simulink model "case4"  (R2024b)
settings: Solver=FixedStepAuto  StartTime=0  StopTime=1  FixedStep=1e-7  RelTol=1e-3
values from neighbouring files (symbols this model uses):
  SG_D_1_D = 0.01056    [IEEE9_case_parameters.m]    (also in case1_parameters.m; case2_parameters.m; case3_parameters.m; case4_parameters.m)
  SG_D_1_EnableSaturation = 0    [IEEE9_case_parameters.m]    (also in case1_parameters.m; case2_parameters.m; case3_parameters.m; case4_parameters.m)
  SG_D_1_f0 = 60    [IEEE9_case_parameters.m]    (also in case1_parameters.m; case2_parameters.m; case3_parameters.m; case4_parameters.m)
  SG_D_1_H = 7.5    [IEEE9_case_parameters.m]    (also in case1_parameters.m; case2_parameters.m; case3_parameters.m; case4_parameters.m)
  SG_D_1_K_A = 20    [IEEE9_case_parameters.m]    (also in case1_parameters.m; case2_parameters.m; case3_parameters.m; case4_parameters.m)
  SG_D_1_K_E = 1.000000e+1    (= 10)    [IEEE9_case_parameters.m]    (also in case1_parameters.m; case2_parameters.m; case3_parameters.m; case4_parameters.m)
  SG_D_1_K_F = 2.363    [IEEE9_case_parameters.m]    (also in case1_parameters.m; case2_parameters.m; case3_parameters.m; case4_parameters.m)
  SG_D_1_K_s = 0.5    [IEEE9_case_parameters.m]    (also in case1_parameters.m = 5; case2_parameters.m = 5; case3_parameters.m = 5; case4_parameters.m = 5)
  SG_D_1_R_a = 0.001088    [IEEE9_case_parameters.m]    (also in case1_parameters.m; case2_parameters.m; case3_parameters.m; case4_parameters.m)
  SG_D_1_S_A = 1    [IEEE9_case_parameters.m]    (also in case1_parameters.m; case2_parameters.m; case3_parameters.m; case4_parameters.m)
  SG_D_1_S_B = 0.103    [IEEE9_case_parameters.m]    (also in case1_parameters.m; case2_parameters.m; case3_parameters.m; case4_parameters.m)
  SG_D_1_S_N = 10.659857    [IEEE9_case_parameters.m]    (also in case1_parameters.m; case2_parameters.m; case3_parameters.m; case4_parameters.m)
  SG_D_1_SpeedPara = 200    [IEEE9_case_parameters.m]    (also in case1_parameters.m; case2_parameters.m; case3_parameters.m; case4_parameters.m)
  SG_D_1_T_0 = 0.720173    [IEEE9_case_parameters.m]    (also in case1_parameters.m = 0.755522; case2_parameters.m = 0.808931; case3_parameters.m = 0.869402; case4_parameters.m = 0.729316)
  SG_D_1_T_1 = 0.3    [IEEE9_case_parameters.m]    (also in case1_parameters.m; case2_parameters.m; case3_parameters.m; case4_parameters.m)
  SG_D_1_T_2 = 0.05    [IEEE9_case_parameters.m]    (also in case1_parameters.m; case2_parameters.m; case3_parameters.m; case4_parameters.m)
  SG_D_1_T_3 = 0.02    [IEEE9_case_parameters.m]    (also in case1_parameters.m; case2_parameters.m; case3_parameters.m; case4_parameters.m)
  SG_D_1_T_4 = 0.005    [IEEE9_case_parameters.m]    (also in case1_parameters.m; case2_parameters.m; case3_parameters.m; case4_parameters.m)
  SG_D_1_T_A = 0.02    [IEEE9_case_parameters.m]    (also in case1_parameters.m; case2_parameters.m; case3_parameters.m; case4_parameters.m)
  SG_D_1_T_dd = 8.000000e+0    (= 8)    [IEEE9_case_parameters.m]    (also in case1_parameters.m; case2_parameters.m; case3_parameters.m; case4_parameters.m)
  SG_D_1_T_ddd = 0.04    [IEEE9_case_parameters.m]    (also in case1_parameters.m; case2_parameters.m; case3_parameters.m; case4_parameters.m)
  SG_D_1_T_E = 0.314    [IEEE9_case_parameters.m]    (also in case1_parameters.m; case2_parameters.m; case3_parameters.m; case4_parameters.m)
  SG_D_1_T_F = 0.35    [IEEE9_case_parameters.m]    (also in case1_parameters.m; case2_parameters.m; case3_parameters.m; case4_parameters.m)
  SG_D_1_T_qd = 0.8    [IEEE9_case_parameters.m]    (also in case1_parameters.m; case2_parameters.m; case3_parameters.m; case4_parameters.m)
  SG_D_1_T_qdd = 0.02    [IEEE9_case_parameters.m]    (also in case1_parameters.m; case2_parameters.m; case3_parameters.m; case4_parameters.m)
  SG_D_1_T_speed = 0.1    [IEEE9_case_parameters.m]    (also in case1_parameters.m = 200; case2_parameters.m = 200; case3_parameters.m = 200; case4_parameters.m = 200)
  SG_D_1_T_w = 0.5    [IEEE9_case_parameters.m]    (also in case1_parameters.m; case2_parameters.m; case3_parameters.m; case4_parameters.m)
  SG_D_1_V_ref = 1.990276    [IEEE9_case_parameters.m]    (also in case1_parameters.m = 2.042296; case2_parameters.m = 2.051388; case3_parameters.m = 2.089584; case4_parameters.m = 2.01845)
  SG_D_1_w_ref = 376.991118    [IEEE9_case_parameters.m]    (also in case1_parameters.m; case2_parameters.m; case3_parameters.m; case4_parameters.m)
  SG_D_1_wb = 6.000000e+1    (= 60)    [IEEE9_case_parameters.m]    (also in case1_parameters.m; case2_parameters.m; case3_parameters.m; case4_parameters.m)
  SG_D_1_x_d = 1.9    [IEEE9_case_parameters.m]    (also in case1_parameters.m; case2_parameters.m; case3_parameters.m; case4_parameters.m)
  SG_D_1_x_dd = 0.302    [IEEE9_case_parameters.m]    (also in case1_parameters.m; case2_parameters.m; case3_parameters.m; case4_parameters.m)
  SG_D_1_x_ddd = 0.204    [IEEE9_case_parameters.m]    (also in case1_parameters.m; case2_parameters.m; case3_parameters.m; case4_parameters.m)
  SG_D_1_x_l = 0.05    [IEEE9_case_parameters.m]    (also in case1_parameters.m; case2_parameters.m; case3_parameters.m; case4_parameters.m)
  SG_D_1_x_q = 1.3    [IEEE9_case_parameters.m]    (also in case1_parameters.m; case2_parameters.m; case3_parameters.m; case4_parameters.m)
  SG_D_1_x_qd = 0.5    [IEEE9_case_parameters.m]    (also in case1_parameters.m; case2_parameters.m; case3_parameters.m; case4_parameters.m)
  SG_D_1_x_qdd = 0.3    [IEEE9_case_parameters.m]    (also in case1_parameters.m; case2_parameters.m; case3_parameters.m; case4_parameters.m)
  SG_D_2_D = 0.02    [IEEE9_case_parameters.m]    (also in case1_parameters.m; case2_parameters.m; case3_parameters.m; case4_parameters.m)
  SG_D_2_EnableSaturation = 0    [IEEE9_case_parameters.m]    (also in case1_parameters.m; case2_parameters.m; case3_parameters.m; case4_parameters.m)
  SG_D_2_f0 = 60    [IEEE9_case_parameters.m]    (also in case1_parameters.m; case2_parameters.m; case3_parameters.m; case4_parameters.m)
  SG_D_2_H = 8.000000e+0    (= 8)    [IEEE9_case_parameters.m]    (also in case1_parameters.m; case2_parameters.m; case3_parameters.m; case4_parameters.m)
  SG_D_2_K_A = 20    [IEEE9_case_parameters.m]    (also in case1_parameters.m; case2_parameters.m; case3_parameters.m; case4_parameters.m)
  SG_D_2_K_E = 1.000000e+1    (= 10)    [IEEE9_case_parameters.m]    (also in case1_parameters.m; case2_parameters.m; case3_parameters.m; case4_parameters.m)
  SG_D_2_K_F = 2.363    [IEEE9_case_parameters.m]    (also in case1_parameters.m; case2_parameters.m; case3_parameters.m; case4_parameters.m)
  SG_D_2_K_s = 0.5    [IEEE9_case_parameters.m]    (also in case1_parameters.m = 4; case2_parameters.m = 4; case3_parameters.m = 4; case4_parameters.m = 4)
  SG_D_2_R_a = 0.001088    [IEEE9_case_parameters.m]    (also in case1_parameters.m; case2_parameters.m; case3_parameters.m; case4_parameters.m)
  SG_D_2_S_A = 1    [IEEE9_case_parameters.m]    (also in case1_parameters.m; case2_parameters.m; case3_parameters.m; case4_parameters.m)
  SG_D_2_S_B = 0.103    [IEEE9_case_parameters.m]    (also in case1_parameters.m; case2_parameters.m; case3_parameters.m; case4_parameters.m)
  SG_D_2_S_N = 10.659857    [IEEE9_case_parameters.m]    (also in case1_parameters.m; case2_parameters.m; case3_parameters.m; case4_parameters.m)
  SG_D_2_SpeedPara = 200    [IEEE9_case_parameters.m]    (also in case1_parameters.m; case2_parameters.m; case3_parameters.m; case4_parameters.m)
  SG_D_2_T_0 = 1.632913    [IEEE9_case_parameters.m]    (also in case1_parameters.m = 1.632925; case2_parameters.m = 1.632915; case3_parameters.m = 1.632914; case4_parameters.m = 1.632927)
  SG_D_2_T_1 = 0.2    [IEEE9_case_parameters.m]    (also in case1_parameters.m; case2_parameters.m; case3_parameters.m; case4_parameters.m)
  SG_D_2_T_2 = 0.05    [IEEE9_case_parameters.m]    (also in case1_parameters.m; case2_parameters.m; case3_parameters.m; case4_parameters.m)
  SG_D_2_T_3 = 0.02    [IEEE9_case_parameters.m]    (also in case1_parameters.m; case2_parameters.m; case3_parameters.m; case4_parameters.m)
  SG_D_2_T_4 = 0.005    [IEEE9_case_parameters.m]    (also in case1_parameters.m; case2_parameters.m; case3_parameters.m; case4_parameters.m)
  SG_D_2_T_A = 0.02    [IEEE9_case_parameters.m]    (also in case1_parameters.m; case2_parameters.m; case3_parameters.m; case4_parameters.m)
  SG_D_2_T_dd = 7.9    [IEEE9_case_parameters.m]    (also in case1_parameters.m; case2_parameters.m; case3_parameters.m; case4_parameters.m)
  SG_D_2_T_ddd = 0.04    [IEEE9_case_parameters.m]    (also in case1_parameters.m; case2_parameters.m; case3_parameters.m; case4_parameters.m)
  SG_D_2_T_E = 0.314    [IEEE9_case_parameters.m]    (also in case1_parameters.m; case2_parameters.m; case3_parameters.m; case4_parameters.m)
  SG_D_2_T_F = 0.35    [IEEE9_case_parameters.m]    (also in case1_parameters.m; case2_parameters.m; case3_parameters.m; case4_parameters.m)
  SG_D_2_T_qd = 0.8    [IEEE9_case_parameters.m]    (also in case1_parameters.m; case2_parameters.m; case3_parameters.m; case4_parameters.m)
  SG_D_2_T_qdd = 0.015    [IEEE9_case_parameters.m]    (also in case1_parameters.m; case2_parameters.m; case3_parameters.m; case4_parameters.m)
  SG_D_2_T_speed = 0.1    [IEEE9_case_parameters.m]    (also in case1_parameters.m = 150; case2_parameters.m = 150; case3_parameters.m = 150; case4_parameters.m = 150)
  SG_D_2_T_w = 0.35    [IEEE9_case_parameters.m]    (also in case1_parameters.m; case2_parameters.m; case3_parameters.m; case4_parameters.m)
  SG_D_2_V_ref = 2.58547    [IEEE9_case_parameters.m]    (also in case1_parameters.m = 2.597896; case2_parameters.m = 2.587136; case3_parameters.m = 2.586042; case4_parameters.m = 2.599679)
  SG_D_2_w_ref = 376.991118    [IEEE9_case_parameters.m]    (also in case1_parameters.m; case2_parameters.m; case3_parameters.m; case4_parameters.m)
  SG_D_2_wb = 6.000000e+1    (= 60)    [IEEE9_case_parameters.m]    (also in case1_parameters.m; case2_parameters.m; case3_parameters.m; case4_parameters.m)
  SG_D_2_x_d = 1.8    [IEEE9_case_parameters.m]    (also in case1_parameters.m; case2_parameters.m; case3_parameters.m; case4_parameters.m)
  SG_D_2_x_dd = 0.302    [IEEE9_case_parameters.m]    (also in case1_parameters.m; case2_parameters.m; case3_parameters.m; case4_parameters.m)
  SG_D_2_x_ddd = 0.204    [IEEE9_case_parameters.m]    (also in case1_parameters.m; case2_parameters.m; case3_parameters.m; case4_parameters.m)
  SG_D_2_x_l = 0.05    [IEEE9_case_parameters.m]    (also in case1_parameters.m; case2_parameters.m; case3_parameters.m; case4_parameters.m)
  SG_D_2_x_q = 1.25    [IEEE9_case_parameters.m]    (also in case1_parameters.m; case2_parameters.m; case3_parameters.m; case4_parameters.m)
  SG_D_2_x_qd = 0.5    [IEEE9_case_parameters.m]    (also in case1_parameters.m; case2_parameters.m; case3_parameters.m; case4_parameters.m)
  SG_D_2_x_qdd = 0.3    [IEEE9_case_parameters.m]    (also in case1_parameters.m; case2_parameters.m; case3_parameters.m; case4_parameters.m)
  SG_D_3_D = 0.02    [IEEE9_case_parameters.m]    (also in case1_parameters.m; case2_parameters.m; case3_parameters.m; case4_parameters.m)
  SG_D_3_EnableSaturation = 0    [IEEE9_case_parameters.m]    (also in case1_parameters.m; case2_parameters.m; case3_parameters.m; case4_parameters.m)
  SG_D_3_f0 = 60    [IEEE9_case_parameters.m]    (also in case1_parameters.m; case2_parameters.m; case3_parameters.m; case4_parameters.m)
  SG_D_3_H = 7.7    [IEEE9_case_parameters.m]    (also in case1_parameters.m; case2_parameters.m; case3_parameters.m; case4_parameters.m)
  SG_D_3_K_A = 20    [IEEE9_case_parameters.m]    (also in case1_parameters.m; case2_parameters.m; case3_parameters.m; case4_parameters.m)
  SG_D_3_K_E = 1.000000e+1    (= 10)    [IEEE9_case_parameters.m]    (also in case1_parameters.m; case2_parameters.m; case3_parameters.m; case4_parameters.m)
  SG_D_3_K_F = 2.363    [IEEE9_case_parameters.m]    (also in case1_parameters.m; case2_parameters.m; case3_parameters.m; case4_parameters.m)
  SG_D_3_K_s = 0.2    [IEEE9_case_parameters.m]    (also in case1_parameters.m = 2; case2_parameters.m = 2; case3_parameters.m = 2; case4_parameters.m = 2)
  SG_D_3_R_a = 0.001088    [IEEE9_case_parameters.m]    (also in case1_parameters.m; case2_parameters.m; case3_parameters.m; case4_parameters.m)
  SG_D_3_S_A = 1    [IEEE9_case_parameters.m]    (also in case1_parameters.m; case2_parameters.m; case3_parameters.m; case4_parameters.m)
  SG_D_3_S_B = 0.103    [IEEE9_case_parameters.m]    (also in case1_parameters.m; case2_parameters.m; case3_parameters.m; case4_parameters.m)
  SG_D_3_S_N = 10.659857    [IEEE9_case_parameters.m]    (also in case1_parameters.m; case2_parameters.m; case3_parameters.m; case4_parameters.m)
  SG_D_3_SpeedPara = 200    [IEEE9_case_parameters.m]    (also in case1_parameters.m; case2_parameters.m; case3_parameters.m; case4_parameters.m)
  SG_D_3_T_0 = 0.850788    [IEEE9_case_parameters.m]    (also in case1_parameters.m = 0.850786; case2_parameters.m = 0.850787; case3_parameters.m; case4_parameters.m = 0.850786)
  SG_D_3_T_1 = 0.2    [IEEE9_case_parameters.m]    (also in case1_parameters.m; case2_parameters.m; case3_parameters.m; case4_parameters.m)
  SG_D_3_T_2 = 0.05    [IEEE9_case_parameters.m]    (also in case1_parameters.m; case2_parameters.m; case3_parameters.m; case4_parameters.m)
  SG_D_3_T_3 = 0.02    [IEEE9_case_parameters.m]    (also in case1_parameters.m; case2_parameters.m; case3_parameters.m; case4_parameters.m)
  SG_D_3_T_4 = 0.005    [IEEE9_case_parameters.m]    (also in case1_parameters.m; case2_parameters.m; case3_parameters.m; case4_parameters.m)
  SG_D_3_T_A = 0.02    [IEEE9_case_parameters.m]    (also in case1_parameters.m; case2_parameters.m; case3_parameters.m; case4_parameters.m)
  SG_D_3_T_dd = 8.1    [IEEE9_case_parameters.m]    (also in case1_parameters.m; case2_parameters.m; case3_parameters.m; case4_parameters.m)
  SG_D_3_T_ddd = 0.04    [IEEE9_case_parameters.m]    (also in case1_parameters.m; case2_parameters.m; case3_parameters.m; case4_parameters.m)
  SG_D_3_T_E = 0.314    [IEEE9_case_parameters.m]    (also in case1_parameters.m; case2_parameters.m; case3_parameters.m; case4_parameters.m)
  SG_D_3_T_F = 0.35    [IEEE9_case_parameters.m]    (also in case1_parameters.m; case2_parameters.m; case3_parameters.m; case4_parameters.m)
  SG_D_3_T_qd = 0.8    [IEEE9_case_parameters.m]    (also in case1_parameters.m; case2_parameters.m; case3_parameters.m; case4_parameters.m)
  SG_D_3_T_qdd = 0.015    [IEEE9_case_parameters.m]    (also in case1_parameters.m; case2_parameters.m; case3_parameters.m; case4_parameters.m)
  SG_D_3_T_speed = 0.1    [IEEE9_case_parameters.m]    (also in case1_parameters.m = 180; case2_parameters.m = 180; case3_parameters.m = 180; case4_parameters.m = 180)
  SG_D_3_T_w = 0.4    [IEEE9_case_parameters.m]    (also in case1_parameters.m; case2_parameters.m; case3_parameters.m; case4_parameters.m)
  SG_D_3_V_ref = 1.892727    [IEEE9_case_parameters.m]    (also in case1_parameters.m = 1.906439; case2_parameters.m = 1.895535; case3_parameters.m = 1.892105; case4_parameters.m = 1.906598)
  SG_D_3_w_ref = 376.991118    [IEEE9_case_parameters.m]    (also in case1_parameters.m; case2_parameters.m; case3_parameters.m; case4_parameters.m)
  SG_D_3_wb = 6.000000e+1    (= 60)    [IEEE9_case_parameters.m]    (also in case1_parameters.m; case2_parameters.m; case3_parameters.m; case4_parameters.m)
  SG_D_3_x_d = 1.85    [IEEE9_case_parameters.m]    (also in case1_parameters.m; case2_parameters.m; case3_parameters.m; case4_parameters.m)
  SG_D_3_x_dd = 0.302    [IEEE9_case_parameters.m]    (also in case1_parameters.m; case2_parameters.m; case3_parameters.m; case4_parameters.m)
  SG_D_3_x_ddd = 0.204    [IEEE9_case_parameters.m]    (also in case1_parameters.m; case2_parameters.m; case3_parameters.m; case4_parameters.m)
  SG_D_3_x_l = 0.05    [IEEE9_case_parameters.m]    (also in case1_parameters.m; case2_parameters.m; case3_parameters.m; case4_parameters.m)
  SG_D_3_x_q = 1.2    [IEEE9_case_parameters.m]    (also in case1_parameters.m; case2_parameters.m; case3_parameters.m; case4_parameters.m)
  SG_D_3_x_qd = 0.5    [IEEE9_case_parameters.m]    (also in case1_parameters.m; case2_parameters.m; case3_parameters.m; case4_parameters.m)
  SG_D_3_x_qdd = 0.3    [IEEE9_case_parameters.m]    (also in case1_parameters.m; case2_parameters.m; case3_parameters.m; case4_parameters.m)
(part 6 of 12)

== system case4/SG_D_1/d_psi_kq_SG_D_1_block ==
  note: d_psi_kq_SG_D_1 in case4
      | $-\frac{\psi _{\mathrm{gq},\mathrm{SG},D,1}+\psi _{\mathrm{kq},\mathrm{SG},D,1}+\frac{\left(x_{l}-x_{\mathrm{qd}}\right)\,\left(\psi _{q,\mathrm{SG},D,1}+\frac{\psi _{\mathrm{gq},\mathrm{SG},D,1}\,\left(x_{l}-x_{\mathrm{qdd}}\right)}{x_{l}-x_{\mathrm{qd}}}+\frac{\psi _{\mathrm{kq},\mathrm{SG},D,1}\,\left(x_{\mathrm{qd}}-x_{\mathrm{qdd}}\right)}{x_{l}-x_{\mathrm{qd}}}\right)}{x_{\mathrm{qdd}}}}{T_{\mathrm{qdd}}}$
      | Automatically generated on 2025-10-31 19:04:27 .
  State_psi_gq_SG_D_1_29a0d : Inport
  State_psi_kq_SG_D_1_bc099 : Inport  Port=2
  State_psi_gq_SG_D_1_826db : Inport  Port=3
  State_psi_kq_SG_D_1_a459f : Inport  Port=4
  State_psi_q_SG_D_1_3b733 : Inport  Port=5
  Add_07a2b : Sum
  Add_0c9f9 : Sum
  Add_8fa00 : Sum
  Add_cf35f : Sum
  Add_e1e4f : Sum
  Add_e3374 : Sum
  Constant_-1_31501 : Constant  Value=-1
  Constant_-1_3fd20 : Constant  Value=-1
  Constant_-1_4f17b : Constant  Value=-1
  Constant_-1_7f992 : Constant  Value=-1
  Constant_-1_cd7b7 : Constant  Value=-1
  Constant_T_qdd_564d8 : Constant  Value=T_qdd
  Constant_x_l_26743 : Constant  Value=x_l
  Constant_x_l_9b9df : Constant  Value=x_l
  Constant_x_l_bfb4c : Constant  Value=x_l
  Constant_x_l_c7950 : Constant  Value=x_l
  Constant_x_qd_1270f : Constant  Value=x_qd
  Constant_x_qd_594fa : Constant  Value=x_qd
  Constant_x_qd_82dbe : Constant  Value=x_qd
  Constant_x_qd_9bdfa : Constant  Value=x_qd
  Constant_x_qdd_52f5f : Constant  Value=x_qdd
  Constant_x_qdd_57218 : Constant  Value=x_qdd
  Constant_x_qdd_a169c : Constant  Value=x_qdd
  Divide_52e8c : Product  Inputs=*/
  Divide_a0622 : Product  Inputs=*/
  Divide_aaa28 : Product  Inputs=*/
  Divide_e46e9 : Product  Inputs=*/
  Product_012aa : Product
  Product_04776 : Product
  Product_0e76a : Product
  Product_19400 : Product
  Product_6a89c : Product
  Product_735d3 : Product
  Product_cfb26 : Product
  Product_d26f0 : Product
  Subtract_17dfd : Sum  Inputs=+-
  Subtract_27213 : Sum  Inputs=+-
  Subtract_9eef0 : Sum  Inputs=+-
  Blockout_d_psi_kq_SG_D_1_c314f : Outport
  wires:
  Product_19400/1 -> Add_0c9f9/1
  Constant_-1_3fd20/1 -> Product_19400/1
  Constant_x_l_c7950/1 -> Product_19400/2
  Constant_x_qdd_a169c/1 -> Add_0c9f9/2
  Constant_-1_4f17b/1 -> Product_735d3/1
  Constant_x_qd_594fa/1 -> Subtract_27213/1
  Constant_x_qd_82dbe/1 -> Add_e1e4f/2
  Constant_-1_cd7b7/1 -> Product_04776/1
  Constant_x_l_9b9df/1 -> Product_735d3/2
  Constant_x_qdd_52f5f/1 -> Subtract_27213/2
  Constant_x_qd_1270f/1 -> Add_e3374/2
  Constant_x_l_bfb4c/1 -> Product_04776/2
  Subtract_9eef0/1 -> Add_07a2b/1
  Product_012aa/1 -> Subtract_9eef0/1
  State_psi_gq_SG_D_1_826db/1 -> Product_6a89c/1
  Add_0c9f9/1 -> Product_6a89c/2
  Product_04776/1 -> Add_8fa00/1
  Constant_x_qd_9bdfa/1 -> Add_8fa00/2
  State_psi_kq_SG_D_1_a459f/1 -> Product_d26f0/1
  Product_735d3/1 -> Add_e3374/1
  Subtract_27213/1 -> Product_d26f0/2
  Product_6a89c/1 -> Divide_52e8c/1
  Add_8fa00/1 -> Divide_52e8c/2
  Product_d26f0/1 -> Divide_e46e9/1
  Add_e3374/1 -> Divide_e46e9/2
  Constant_-1_7f992/1 -> Product_cfb26/1
  Constant_x_l_26743/1 -> Product_cfb26/2
  Divide_52e8c/1 -> Subtract_17dfd/1
  Divide_e46e9/1 -> Subtract_17dfd/2
  Product_cfb26/1 -> Add_e1e4f/1
  Add_cf35f/1 -> Product_0e76a/2
  Subtract_17dfd/1 -> Add_cf35f/1
  State_psi_q_SG_D_1_3b733/1 -> Add_cf35f/2
  Constant_-1_31501/1 -> Product_012aa/1
  State_psi_gq_SG_D_1_29a0d/1 -> Product_012aa/2
  Divide_a0622/1 -> Add_07a2b/2
  Product_0e76a/1 -> Divide_a0622/1
  Add_e1e4f/1 -> Product_0e76a/1
  State_psi_kq_SG_D_1_bc099/1 -> Subtract_9eef0/2
  Constant_x_qdd_57218/1 -> Divide_a0622/2
  Add_07a2b/1 -> Divide_aaa28/1
  Constant_T_qdd_564d8/1 -> Divide_aaa28/2
  Divide_aaa28/1 -> Blockout_d_psi_kq_SG_D_1_c314f/1

== system case4/SG_D_1/d_psi_q_SG_D_1_block ==
  note: d_psi_q_SG_D_1 in case4
      | $2\,\pi \,f_{0}\,\left(v_{d,\mathrm{SG},D,1}\,\cos\left(\theta _{\mathrm{SG},D,1}\right)+v_{q,\mathrm{SG},D,1}\,\sin\left(\theta _{\mathrm{SG},D,1}\right)-\frac{R_{a}\,\left(\psi _{q,\mathrm{SG},D,1}+\frac{\psi _{\mathrm{gq},\mathrm{SG},D,1}\,\left(x_{l}-x_{\mathrm{qdd}}\right)}{x_{l}-x_{\mathrm{qd}}}+\frac{\psi _{\mathrm{kq},\mathrm{SG},D,1}\,\left(x_{\mathrm{qd}}-x_{\mathrm{qdd}}\right)}{x_{l}-x_{\mathrm{qd}}}\right)}{x_{\mathrm{qdd}}}-\frac{\psi _{d,\mathrm{SG},D,1}\,w_{\mathrm{SG},D,1}}{2\,f_{0}\,\pi }\right)$
      | Automatically generated on 2025-10-31 19:04:10 .
  State_psi_gq_SG_D_1_fb8d0 : Inport
  State_psi_kq_SG_D_1_6d221 : Inport  Port=2
  State_psi_q_SG_D_1_4ef79 : Inport  Port=3
  Input_v_d_SG_D_1_90d90 : Inport  Port=4
  State_theta_SG_D_1_b8399 : Inport  Port=5
  Input_v_q_SG_D_1_a80c5 : Inport  Port=6
  State_theta_SG_D_1_5aa7f : Inport  Port=7
  State_psi_d_SG_D_1_9f1e2 : Inport  Port=8
  State_w_SG_D_1_ddf4d : Inport  Port=9
  Add_0c463 : Sum
  Add_8a4b3 : Sum
  Add_912f8 : Sum
  Add_b64c2 : Sum
  Add_ef9af : Sum
  Constant_-1_80688 : Constant  Value=-1
  Constant_-1_b4c60 : Constant  Value=-1
  Constant_-1_cea76 : Constant  Value=-1
  Constant_-2.0_e970a : Constant  Value=-2.0
  Constant_2.0_e1228 : Constant  Value=2.0
  Constant_R_a_03999 : Constant  Value=R_a
  Constant_f0_4ffcb : Constant  Value=f0
  Constant_f0_905ff : Constant  Value=f0
  Constant_pi_9b720 : Constant  Value=pi
  Constant_pi_d0bc2 : Constant  Value=pi
  Constant_x_l_53855 : Constant  Value=x_l
  Constant_x_l_53897 : Constant  Value=x_l
  Constant_x_l_83613 : Constant  Value=x_l
  Constant_x_qd_3e080 : Constant  Value=x_qd
  Constant_x_qd_9aab5 : Constant  Value=x_qd
  Constant_x_qd_afd52 : Constant  Value=x_qd
  Constant_x_qdd_29a16 : Constant  Value=x_qdd
  Constant_x_qdd_e01f0 : Constant  Value=x_qdd
  Constant_x_qdd_f701c : Constant  Value=x_qdd
  Divide_05d1f : Product  Inputs=*/
  Divide_4fc8e : Product  Inputs=*/
  Divide_af232 : Product  Inputs=*/
  Divide_f9f99 : Product  Inputs=*/
  MathFunc_cos_74157 : Trigonometry  Operator=cos
  MathFunc_sin_8c450 : Trigonometry
  Product_00d40 : Product
  Product_07fa6 : Product
  Product_09192 : Product
  Product_26fa1 : Product
  Product_29f0a : Product
  Product_4895a : Product
  Product_4d44b : Product
  Product_53177 : Product
  Product_5f087 : Product
  Product_64f31 : Product
  Product_70c29 : Product
  Product_acc0c : Product
  Product_bb502 : Product
  Product_e5a33 : Product
  Subtract_24f23 : Sum  Inputs=+-
  Subtract_3197c : Sum  Inputs=+-
  Subtract_ca882 : Sum  Inputs=+-
  Subtract_fa220 : Sum  Inputs=+-
  Blockout_d_psi_q_SG_D_1_390c6 : Outport
  wires:
  Divide_af232/1 -> Subtract_fa220/1
  Product_acc0c/1 -> Add_912f8/1
  Constant_x_l_83613/1 -> Product_acc0c/2
  Constant_-1_cea76/1 -> Product_acc0c/1
  Constant_x_qdd_29a16/1 -> Add_912f8/2
  Constant_x_l_53855/1 -> Product_00d40/2
  Constant_-1_b4c60/1 -> Product_00d40/1
  Constant_x_l_53897/1 -> Product_4895a/2
  Constant_x_qdd_e01f0/1 -> Subtract_ca882/2
  State_psi_kq_SG_D_1_6d221/1 -> Product_53177/1
  Constant_-1_80688/1 -> Product_4895a/1
  Constant_x_qd_3e080/1 -> Subtract_ca882/1
  State_psi_gq_SG_D_1_fb8d0/1 -> Product_64f31/1
  Product_07fa6/1 -> Blockout_d_psi_q_SG_D_1_390c6/1
  Subtract_fa220/1 -> Add_ef9af/1
  Product_64f31/1 -> Divide_af232/1
  Add_912f8/1 -> Product_64f31/2
  Divide_05d1f/1 -> Subtract_fa220/2
  Product_00d40/1 -> Add_8a4b3/1
  Constant_x_qd_afd52/1 -> Add_8a4b3/2
  Constant_-2.0_e970a/1 -> Product_bb502/1
  Product_53177/1 -> Divide_05d1f/1
  Product_4895a/1 -> Add_b64c2/1
  Subtract_ca882/1 -> Product_53177/2
  Constant_x_qd_9aab5/1 -> Add_b64c2/2
  Add_8a4b3/1 -> Divide_af232/2
  Add_b64c2/1 -> Divide_05d1f/2
  Constant_f0_905ff/1 -> Product_26fa1/2
  State_psi_q_SG_D_1_4ef79/1 -> Add_ef9af/2
  Product_e5a33/1 -> Product_4d44b/1
  Constant_R_a_03999/1 -> Product_70c29/1
  Product_4d44b/1 -> Divide_f9f99/2
  Product_70c29/1 -> Divide_4fc8e/1
  Add_ef9af/1 -> Product_70c29/2
  State_theta_SG_D_1_b8399/1 -> MathFunc_cos_74157/1
  Input_v_d_SG_D_1_90d90/1 -> Product_29f0a/1
  Constant_x_qdd_f701c/1 -> Divide_4fc8e/2
  MathFunc_cos_74157/1 -> Product_29f0a/2
  State_theta_SG_D_1_5aa7f/1 -> MathFunc_sin_8c450/1
  Divide_4fc8e/1 -> Subtract_24f23/1
  Constant_2.0_e1228/1 -> Product_e5a33/1
  State_w_SG_D_1_ddf4d/1 -> Product_09192/2
  Constant_pi_9b720/1 -> Product_e5a33/2
  Subtract_3197c/1 -> Add_0c463/1
  Product_29f0a/1 -> Subtract_24f23/2
  Divide_f9f99/1 -> Add_0c463/2
  Input_v_q_SG_D_1_a80c5/1 -> Product_5f087/1
  MathFunc_sin_8c450/1 -> Product_5f087/2
  Product_5f087/1 -> Subtract_3197c/2
  State_psi_d_SG_D_1_9f1e2/1 -> Product_09192/1
  Constant_f0_4ffcb/1 -> Product_4d44b/2
  Constant_pi_d0bc2/1 -> Product_bb502/2
  Subtract_24f23/1 -> Subtract_3197c/1
  Product_09192/1 -> Divide_f9f99/1
  Product_bb502/1 -> Product_26fa1/1
  Product_26fa1/1 -> Product_07fa6/1
  Add_0c463/1 -> Product_07fa6/2

== system case4/SG_D_1/d_theta_SG_D_1_block ==
  note: d_theta_SG_D_1 in case4
      | $w_{\mathrm{SG},D,1}-2\,\pi \,f_{0}$
      | Automatically generated on 2025-10-31 19:04:34 .
  State_w_SG_D_1_f434c : Inport
  Add_da730 : Sum
  Constant_-2.0_5dbd2 : Constant  Value=-2.0
  Constant_f0_d77fd : Constant  Value=f0
  Constant_pi_88a66 : Constant  Value=pi
  Product_1a1b7 : Product
  Product_ddc24 : Product
  Blockout_d_theta_SG_D_1_0ea3b : Outport
  wires:
  State_w_SG_D_1_f434c/1 -> Add_da730/2
  Constant_-2.0_5dbd2/1 -> Product_ddc24/1
  Constant_f0_d77fd/1 -> Product_1a1b7/2
  Constant_pi_88a66/1 -> Product_ddc24/2
  Product_1a1b7/1 -> Add_da730/1
  Product_ddc24/1 -> Product_1a1b7/1
  Add_da730/1 -> Blockout_d_theta_SG_D_1_0ea3b/1

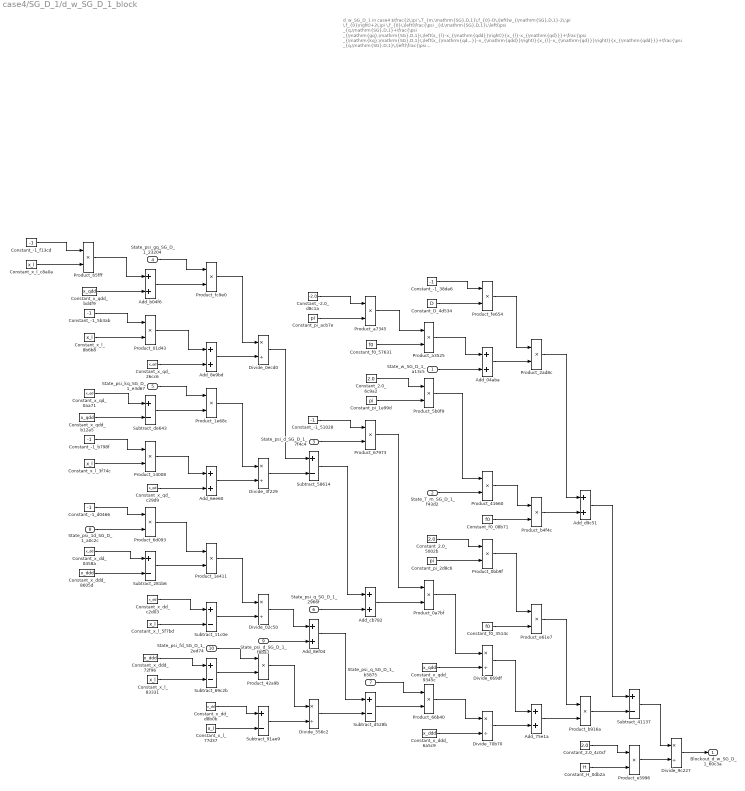
== system case4/SG_D_1/d_w_SG_D_1_block ==
  note: d_w_SG_D_1 in case4
      | $\frac{2\,\pi \,T_{m,\mathrm{SG},D,1}\,f_{0}-D\,\left(w_{\mathrm{SG},D,1}-2\,\pi \,f_{0}\right)+2\,\pi \,f_{0}\,\left(\frac{\psi _{d,\mathrm{SG},D,1}\,\left(\psi _{q,\mathrm{SG},D,1}+\frac{\psi _{\mathrm{gq},\mathrm{SG},D,1}\,\left(x_{l}-x_{\mathrm{qdd}}\right)}{x_{l}-x_{\mathrm{qd}}}+\frac{\psi _{\mathrm{kq},\mathrm{SG},D,1}\,\left(x_{\mathrm{qd}}-x_{\mathrm{qdd}}\right)}{x_{l}-x_{\mathrm{qd}}}\right)}{x_{\mathrm{qdd}}}+\frac{\psi _{q,\mathrm{SG},D,1}\,\left(\frac{\psi _{\mathrm{1d},\mathrm{SG},D,1}\,\left(x_{\mathrm{dd}}-x_{\mathrm{ddd}}\right)}{x_{\mathrm{dd}}-x_{l}}-\psi _{d,\mathrm{SG},D,1}+\frac{\psi _{\mathrm{fd},\mathrm{SG},D,1}\,\left(x_{\mathrm{ddd}}-x_{l}\right)}{x_{\mathrm{dd}}-x_{l}}\right)}{x_{\mathrm{ddd}}}\right)}{2\,H}$
      | Automatically generated on 2025-10-31 19:04:33 .
  State_w_SG_D_1_a13c5 : Inport
  State_T_m_SG_D_1_f43d2 : Inport  Port=2
  State_psi_d_SG_D_1_7f4c4 : Inport  Port=3
  State_psi_gq_SG_D_1_23204 : Inport  Port=4
  State_psi_kq_SG_D_1_e3d67 : Inport  Port=5
  State_psi_q_SG_D_1_2966f : Inport  Port=6
  State_psi_q_SG_D_1_b5875 : Inport  Port=7
  State_psi_1d_SG_D_1_a0c2c : Inport  Port=8
  State_psi_d_SG_D_1_f8ba7 : Inport  Port=9
  State_psi_fd_SG_D_1_2ed74 : Inport  Port=10
  Add_04aba : Sum
  Add_6ee60 : Sum
  Add_75e1a : Sum
  Add_8e9bd : Sum
  Add_8ef04 : Sum
  Add_b04f6 : Sum
  Add_cb782 : Sum
  Add_d9c51 : Sum
  Constant_-1_38da6 : Constant  Value=-1
  Constant_-1_51028 : Constant  Value=-1
  Constant_-1_5b3ab : Constant  Value=-1
  Constant_-1_b798f : Constant  Value=-1
  Constant_-1_d0466 : Constant  Value=-1
  Constant_-1_f13cd : Constant  Value=-1
  Constant_-2.0_d8c1a : Constant  Value=-2.0
  Constant_2.0_4c0cf : Constant  Value=2.0
  Constant_2.0_5002b : Constant  Value=2.0
  Constant_2.0_6c9a2 : Constant  Value=2.0
  Constant_D_4d534 : Constant  Value=D
  Constant_H_0db2a : Constant  Value=H
  Constant_f0_08b71 : Constant  Value=f0
  Constant_f0_3514c : Constant  Value=f0
  Constant_f0_57631 : Constant  Value=f0
  Constant_pi_1e99d : Constant  Value=pi
  Constant_pi_2d8c6 : Constant  Value=pi
  Constant_pi_acb7e : Constant  Value=pi
  Constant_x_dd_0458a : Constant  Value=x_dd
  Constant_x_dd_c2d03 : Constant  Value=x_dd
  Constant_x_dd_d8b0b : Constant  Value=x_dd
  Constant_x_ddd_6a5c9 : Constant  Value=x_ddd
  Constant_x_ddd_72f96 : Constant  Value=x_ddd
  Constant_x_ddd_8605d : Constant  Value=x_ddd
  Constant_x_l_3f74c : Constant  Value=x_l
  Constant_x_l_5f7bd : Constant  Value=x_l
  Constant_x_l_77d37 : Constant  Value=x_l
  Constant_x_l_83331 : Constant  Value=x_l
  Constant_x_l_8b6b8 : Constant  Value=x_l
  Constant_x_l_c8a0a : Constant  Value=x_l
  Constant_x_qd_0aa71 : Constant  Value=x_qd
  Constant_x_qd_26cc6 : Constant  Value=x_qd
  Constant_x_qd_c29d9 : Constant  Value=x_qd
  Constant_x_qdd_9345c : Constant  Value=x_qdd
  Constant_x_qdd_b12a5 : Constant  Value=x_qdd
  Constant_x_qdd_bd4f9 : Constant  Value=x_qdd
  Divide_02c50 : Product  Inputs=*/
  Divide_0ecd0 : Product  Inputs=*/
  Divide_3f229 : Product  Inputs=*/
  Divide_556c2 : Product  Inputs=*/
  Divide_669df : Product  Inputs=*/
  Divide_70b70 : Product  Inputs=*/
  Divide_9c227 : Product  Inputs=*/
  Product_01d43 : Product
  Product_0a7bf : Product
  Product_0bb9f : Product
  Product_14008 : Product
  Product_1e411 : Product
  Product_1e68c : Product
  Product_2ad8c : Product
  Product_41660 : Product
  Product_42a9b : Product
  Product_5b0f9 : Product
  Product_65fff : Product
  Product_66b40 : Product
  Product_67973 : Product
  Product_6d093 : Product
  Product_a3525 : Product
  Product_a7345 : Product
  Product_b4f4c : Product
  Product_b916a : Product
  Product_e5996 : Product
  Product_e61e7 : Product
  Product_fc9e0 : Product
  Product_fe654 : Product
  Subtract_11c0e : Sum  Inputs=+-
  Subtract_281b6 : Sum  Inputs=+-
  Subtract_41137 : Sum  Inputs=+-
  Subtract_58614 : Sum  Inputs=+-
  Subtract_69c2b : Sum  Inputs=+-
  Subtract_91ae9 : Sum  Inputs=+-
  Subtract_d528b : Sum  Inputs=+-
  Subtract_de643 : Sum  Inputs=+-
  Blockout_d_w_SG_D_1_60c3a : Outport
  wires:
  Product_a3525/1 -> Add_04aba/1
  Constant_-1_f13cd/1 -> Product_65fff/1
  Constant_pi_1e99d/1 -> Product_5b0f9/2
  Constant_x_qdd_bd4f9/1 -> Add_b04f6/2
  Constant_x_l_c8a0a/1 -> Product_65fff/2
  Product_65fff/1 -> Add_b04f6/1
  Constant_x_qd_0aa71/1 -> Subtract_de643/1
  Constant_-1_5b3ab/1 -> Product_01d43/1
  Product_a7345/1 -> Product_a3525/1
  Constant_x_qdd_b12a5/1 -> Subtract_de643/2
  State_psi_q_SG_D_1_b5875/1 -> Product_66b40/1
  Constant_x_l_8b6b8/1 -> Product_01d43/2
  Constant_-1_b798f/1 -> Product_14008/1
  Constant_x_l_3f74c/1 -> Product_14008/2
  Constant_-1_d0466/1 -> Product_6d093/1
  Product_01d43/1 -> Add_8e9bd/1
  State_psi_1d_SG_D_1_a0c2c/1 -> Product_6d093/2
  Constant_x_dd_0458a/1 -> Subtract_281b6/1
  Subtract_de643/1 -> Product_1e68c/2
  Constant_x_ddd_8605d/1 -> Subtract_281b6/2
  State_psi_gq_SG_D_1_23204/1 -> Product_fc9e0/1
  Product_67973/1 -> Product_0a7bf/1
  Add_b04f6/1 -> Product_fc9e0/2
  Constant_x_qd_26cc6/1 -> Add_8e9bd/2
  State_psi_kq_SG_D_1_e3d67/1 -> Product_1e68c/1
  Constant_f0_57631/1 -> Product_a3525/2
  Product_14008/1 -> Add_6ee60/1
  Constant_x_dd_c2d03/1 -> Subtract_11c0e/1
  Constant_x_qd_c29d9/1 -> Add_6ee60/2
  Product_6d093/1 -> Product_1e411/1
  Subtract_281b6/1 -> Product_1e411/2
  Constant_x_l_5f7bd/1 -> Subtract_11c0e/2
  Constant_x_ddd_72f96/1 -> Subtract_69c2b/1
  Constant_x_l_83331/1 -> Subtract_69c2b/2
  State_w_SG_D_1_a13c5/1 -> Add_04aba/2
  Divide_669df/1 -> Add_75e1a/1
  Constant_-1_38da6/1 -> Product_fe654/1
  Product_fc9e0/1 -> Divide_0ecd0/1
  Add_04aba/1 -> Product_2ad8c/2
  Divide_0ecd0/1 -> Subtract_58614/1
  Add_8e9bd/1 -> Divide_0ecd0/2
  Constant_pi_acb7e/1 -> Product_a7345/2
  Product_1e68c/1 -> Divide_3f229/1
  Add_6ee60/1 -> Divide_3f229/2
  Product_1e411/1 -> Divide_02c50/1
  Divide_02c50/1 -> Add_8ef04/1
  Subtract_11c0e/1 -> Divide_02c50/2
  State_psi_fd_SG_D_1_2ed74/1 -> Product_42a9b/1
  Subtract_69c2b/1 -> Product_42a9b/2
  Constant_x_dd_d8b0b/1 -> Subtract_91ae9/1
  Constant_x_l_77d37/1 -> Subtract_91ae9/2
  Divide_3f229/1 -> Subtract_58614/2
  Constant_2.0_6c9a2/1 -> Product_5b0f9/1
  State_psi_d_SG_D_1_f8ba7/1 -> Add_8ef04/2
  Product_42a9b/1 -> Divide_556c2/1
  Subtract_91ae9/1 -> Divide_556c2/2
  Constant_-2.0_d8c1a/1 -> Product_a7345/1
  Constant_-1_51028/1 -> Product_67973/1
  State_psi_d_SG_D_1_7f4c4/1 -> Product_67973/2
  Subtract_58614/1 -> Add_cb782/1
  Subtract_d528b/1 -> Product_66b40/2
  State_psi_q_SG_D_1_2966f/1 -> Add_cb782/2
  Add_8ef04/1 -> Subtract_d528b/1
  Divide_556c2/1 -> Subtract_d528b/2
  Add_cb782/1 -> Product_0a7bf/2
  Constant_D_4d534/1 -> Product_fe654/2
  Product_5b0f9/1 -> Product_41660/1
  State_T_m_SG_D_1_f43d2/1 -> Product_41660/2
  Constant_2.0_5002b/1 -> Product_0bb9f/1
  Constant_pi_2d8c6/1 -> Product_0bb9f/2
  Product_0a7bf/1 -> Divide_669df/1
  Constant_x_qdd_9345c/1 -> Divide_669df/2
  Product_66b40/1 -> Divide_70b70/1
  Constant_x_ddd_6a5c9/1 -> Divide_70b70/2
  Product_fe654/1 -> Product_2ad8c/1
  Product_41660/1 -> Product_b4f4c/1
  Constant_f0_08b71/1 -> Product_b4f4c/2
  Product_0bb9f/1 -> Product_e61e7/1
  Constant_f0_3514c/1 -> Product_e61e7/2
  Divide_70b70/1 -> Add_75e1a/2
  Product_2ad8c/1 -> Add_d9c51/1
  Product_b4f4c/1 -> Add_d9c51/2
  Product_e61e7/1 -> Product_b916a/1
  Add_75e1a/1 -> Product_b916a/2
  Add_d9c51/1 -> Subtract_41137/1
  Product_b916a/1 -> Subtract_41137/2
  Constant_2.0_4c0cf/1 -> Product_e5996/1
  Constant_H_0db2a/1 -> Product_e5996/2
  Subtract_41137/1 -> Divide_9c227/1
  Product_e5996/1 -> Divide_9c227/2
  Divide_9c227/1 -> Blockout_d_w_SG_D_1_60c3a/1

== system case4/SG_D_1/i_d_SG_D_1_block ==
  note: i_d_SG_D_1 in case4
      | $\frac{\sin\left(\theta _{\mathrm{SG},D,1}\right)\,\left(\frac{\psi _{\mathrm{1d},\mathrm{SG},D,1}\,\left(x_{\mathrm{dd}}-x_{\mathrm{ddd}}\right)}{x_{\mathrm{dd}}-x_{l}}-\psi _{d,\mathrm{SG},D,1}+\frac{\psi _{\mathrm{fd},\mathrm{SG},D,1}\,\left(x_{\mathrm{ddd}}-x_{l}\right)}{x_{\mathrm{dd}}-x_{l}}\right)}{x_{\mathrm{ddd}}}-\frac{\cos\left(\theta _{\mathrm{SG},D,1}\right)\,\left(\psi _{q,\mathrm{SG},D,1}+\frac{\psi _{\mathrm{gq},\mathrm{SG},D,1}\,\left(x_{l}-x_{\mathrm{qdd}}\right)}{x_{l}-x_{\mathrm{qd}}}+\frac{\psi _{\mathrm{kq},\mathrm{SG},D,1}\,\left(x_{\mathrm{qd}}-x_{\mathrm{qdd}}\right)}{x_{l}-x_{\mathrm{qd}}}\right)}{x_{\mathrm{qdd}}}$
      | Automatically generated on 2025-10-31 19:04:54 .
  State_psi_gq_SG_D_1_d0d2e : Inport
  State_psi_kq_SG_D_1_27fd3 : Inport  Port=2
  State_psi_q_SG_D_1_7ff6d : Inport  Port=3
  State_theta_SG_D_1_c0d2f : Inport  Port=4
  State_psi_1d_SG_D_1_c944b : Inport  Port=5
  State_psi_d_SG_D_1_499ff : Inport  Port=6
  State_psi_fd_SG_D_1_cd963 : Inport  Port=7
  State_theta_SG_D_1_3521f : Inport  Port=8
  Add_1f7f8 : Sum
  Add_7156b : Sum
  Add_9420b : Sum
  Add_9af70 : Sum
  Add_e2455 : Sum
  Constant_-1_23de9 : Constant  Value=-1
  Constant_-1_2ec58 : Constant  Value=-1
  Constant_-1_3c751 : Constant  Value=-1
  Constant_-1_74171 : Constant  Value=-1
  Constant_-1_b4175 : Constant  Value=-1
  Constant_x_dd_394ca : Constant  Value=x_dd
  Constant_x_dd_4bd80 : Constant  Value=x_dd
  Constant_x_dd_85148 : Constant  Value=x_dd
  Constant_x_ddd_2bff3 : Constant  Value=x_ddd
  Constant_x_ddd_8275b : Constant  Value=x_ddd
  Constant_x_ddd_98c3b : Constant  Value=x_ddd
  Constant_x_l_0c7a7 : Constant  Value=x_l
  Constant_x_l_33219 : Constant  Value=x_l
  Constant_x_l_39fa4 : Constant  Value=x_l
  Constant_x_l_424f5 : Constant  Value=x_l
  Constant_x_l_5794e : Constant  Value=x_l
  Constant_x_l_d9610 : Constant  Value=x_l
  Constant_x_qd_3c50d : Constant  Value=x_qd
  Constant_x_qd_a3809 : Constant  Value=x_qd
  Constant_x_qd_aebdf : Constant  Value=x_qd
  Constant_x_qdd_4156e : Constant  Value=x_qdd
  Constant_x_qdd_5d381 : Constant  Value=x_qdd
  Constant_x_qdd_dc6aa : Constant  Value=x_qdd
  Divide_51f36 : Product  Inputs=*/
  Divide_7b165 : Product  Inputs=*/
  Divide_9f203 : Product  Inputs=*/
  Divide_ca9f2 : Product  Inputs=*/
  Divide_d64de : Product  Inputs=*/
  Divide_fcbde : Product  Inputs=*/
  MathFunc_cos_88a19 : Trigonometry  Operator=cos
  MathFunc_sin_f2c1c : Trigonometry
  Product_0021f : Product
  Product_08082 : Product
  Product_28a43 : Product
  Product_2e6eb : Product
  Product_39b66 : Product
  Product_48efb : Product
  Product_4d9aa : Product
  Product_7f12d : Product
  Product_87112 : Product
  Product_dc687 : Product
  Product_fbca7 : Product
  Subtract_07f09 : Sum  Inputs=+-
  Subtract_1d7cf : Sum  Inputs=+-
  Subtract_489aa : Sum  Inputs=+-
  Subtract_4e1d7 : Sum  Inputs=+-
  Subtract_84987 : Sum  Inputs=+-
  Subtract_8f64e : Sum  Inputs=+-
  Subtract_cdc70 : Sum  Inputs=+-
  Subtract_f6d43 : Sum  Inputs=+-
  Blockout_i_d_SG_D_1_645b0 : Outport
  wires:
  Constant_-1_3c751/1 -> Product_08082/1
  Constant_x_l_39fa4/1 -> Product_08082/2
  Constant_x_ddd_2bff3/1 -> Subtract_cdc70/2
  Product_08082/1 -> Add_9af70/1
  Constant_x_qdd_4156e/1 -> Subtract_07f09/2
  Constant_x_l_33219/1 -> Product_2e6eb/2
  Constant_x_qd_aebdf/1 -> Add_1f7f8/2
  Constant_x_qdd_dc6aa/1 -> Add_9af70/2
  Constant_x_qd_3c50d/1 -> Subtract_07f09/1
  MathFunc_cos_88a19/1 -> Product_48efb/2
  Constant_-1_b4175/1 -> Product_2e6eb/1
  Constant_-1_23de9/1 -> Product_28a43/1
  Subtract_1d7cf/1 -> Blockout_i_d_SG_D_1_645b0/1
  Constant_x_l_d9610/1 -> Product_28a43/2
  Divide_fcbde/1 -> Subtract_4e1d7/1
  State_psi_gq_SG_D_1_d0d2e/1 -> Product_fbca7/1
  Subtract_489aa/1 -> Product_4d9aa/2
  Add_9af70/1 -> Product_fbca7/2
  Divide_9f203/1 -> Add_9420b/1
  Product_2e6eb/1 -> Add_e2455/1
  Constant_x_qd_a3809/1 -> Add_e2455/2
  State_psi_kq_SG_D_1_27fd3/1 -> Product_dc687/1
  Add_9420b/1 -> Subtract_84987/1
  Add_e2455/1 -> Divide_fcbde/2
  Subtract_07f09/1 -> Product_dc687/2
  Product_28a43/1 -> Add_1f7f8/1
  Constant_-1_2ec58/1 -> Product_39b66/1
  State_psi_1d_SG_D_1_c944b/1 -> Product_39b66/2
  Constant_x_dd_394ca/1 -> Subtract_cdc70/1
  Product_fbca7/1 -> Divide_fcbde/1
  Product_7f12d/1 -> Divide_ca9f2/1
  Subtract_cdc70/1 -> Product_0021f/2
  Product_dc687/1 -> Divide_51f36/1
  Product_39b66/1 -> Product_0021f/1
  Add_1f7f8/1 -> Divide_51f36/2
  Constant_x_dd_4bd80/1 -> Subtract_f6d43/1
  Subtract_4e1d7/1 -> Add_7156b/1
  Constant_x_l_424f5/1 -> Subtract_f6d43/2
  Constant_x_ddd_8275b/1 -> Subtract_489aa/1
  Constant_x_l_5794e/1 -> Subtract_489aa/2
  Divide_ca9f2/1 -> Subtract_1d7cf/2
  Divide_51f36/1 -> Subtract_4e1d7/2
  State_theta_SG_D_1_c0d2f/1 -> MathFunc_cos_88a19/1
  Product_0021f/1 -> Divide_9f203/1
  Subtract_f6d43/1 -> Divide_9f203/2
  State_theta_SG_D_1_3521f/1 -> MathFunc_sin_f2c1c/1
  State_psi_fd_SG_D_1_cd963/1 -> Product_4d9aa/1
  Constant_x_dd_85148/1 -> Subtract_8f64e/1
  Constant_x_l_0c7a7/1 -> Subtract_8f64e/2
  State_psi_q_SG_D_1_7ff6d/1 -> Add_7156b/2
  State_psi_d_SG_D_1_499ff/1 -> Add_9420b/2
  Constant_x_ddd_98c3b/1 -> Divide_ca9f2/2
  MathFunc_sin_f2c1c/1 -> Product_7f12d/2
  Product_4d9aa/1 -> Divide_d64de/1
  Constant_-1_74171/1 -> Product_87112/1
  Subtract_8f64e/1 -> Divide_d64de/2
  Add_7156b/1 -> Product_87112/2
  Divide_d64de/1 -> Subtract_84987/2
  Product_87112/1 -> Product_48efb/1
  Subtract_84987/1 -> Product_7f12d/1
  Constant_x_qdd_5d381/1 -> Divide_7b165/2
  Product_48efb/1 -> Divide_7b165/1
  Divide_7b165/1 -> Subtract_1d7cf/1

== system case4/SG_D_1/i_q_SG_D_1_block ==
  note: i_q_SG_D_1 in case4
      | $-\frac{\sin\left(\theta _{\mathrm{SG},D,1}\right)\,\left(\psi _{q,\mathrm{SG},D,1}+\frac{\psi _{\mathrm{gq},\mathrm{SG},D,1}\,\left(x_{l}-x_{\mathrm{qdd}}\right)}{x_{l}-x_{\mathrm{qd}}}+\frac{\psi _{\mathrm{kq},\mathrm{SG},D,1}\,\left(x_{\mathrm{qd}}-x_{\mathrm{qdd}}\right)}{x_{l}-x_{\mathrm{qd}}}\right)}{x_{\mathrm{qdd}}}-\frac{\cos\left(\theta _{\mathrm{SG},D,1}\right)\,\left(\frac{\psi _{\mathrm{1d},\mathrm{SG},D,1}\,\left(x_{\mathrm{dd}}-x_{\mathrm{ddd}}\right)}{x_{\mathrm{dd}}-x_{l}}-\psi _{d,\mathrm{SG},D,1}+\frac{\psi _{\mathrm{fd},\mathrm{SG},D,1}\,\left(x_{\mathrm{ddd}}-x_{l}\right)}{x_{\mathrm{dd}}-x_{l}}\right)}{x_{\mathrm{ddd}}}$
      | Automatically generated on 2025-10-31 19:04:57 .
  State_psi_gq_SG_D_1_2717f : Inport
  State_psi_kq_SG_D_1_bf4f0 : Inport  Port=2
  State_psi_q_SG_D_1_74a75 : Inport  Port=3
  State_theta_SG_D_1_baa8c : Inport  Port=4
  State_psi_1d_SG_D_1_d0628 : Inport  Port=5
  State_psi_d_SG_D_1_d0c9d : Inport  Port=6
  State_psi_fd_SG_D_1_58d0e : Inport  Port=7
  State_theta_SG_D_1_20748 : Inport  Port=8
  Add_179e8 : Sum
  Add_2e471 : Sum
  Add_a0598 : Sum
  Add_a475c : Sum
  Add_ee79c : Sum
  Add_f0bd1 : Sum
  Constant_-1_3d43a : Constant  Value=-1
  Constant_-1_41cb1 : Constant  Value=-1
  Constant_-1_715c3 : Constant  Value=-1
  Constant_-1_8e5d6 : Constant  Value=-1
  Constant_-1_a70be : Constant  Value=-1
  Constant_x_dd_5089f : Constant  Value=x_dd
  Constant_x_dd_bd8fd : Constant  Value=x_dd
  Constant_x_dd_fe5f8 : Constant  Value=x_dd
  Constant_x_ddd_2672a : Constant  Value=x_ddd
  Constant_x_ddd_50ed9 : Constant  Value=x_ddd
  Constant_x_ddd_523dc : Constant  Value=x_ddd
  Constant_x_l_111e7 : Constant  Value=x_l
  Constant_x_l_3aa63 : Constant  Value=x_l
  Constant_x_l_46464 : Constant  Value=x_l
  Constant_x_l_6df76 : Constant  Value=x_l
  Constant_x_l_81982 : Constant  Value=x_l
  Constant_x_l_cee03 : Constant  Value=x_l
  Constant_x_qd_4819b : Constant  Value=x_qd
  Constant_x_qd_d5e1f : Constant  Value=x_qd
  Constant_x_qd_f127c : Constant  Value=x_qd
  Constant_x_qdd_04085 : Constant  Value=x_qdd
  Constant_x_qdd_0f738 : Constant  Value=x_qdd
  Constant_x_qdd_325a0 : Constant  Value=x_qdd
  Divide_2e8ec : Product  Inputs=*/
  Divide_58af2 : Product  Inputs=*/
  Divide_663fd : Product  Inputs=*/
  Divide_86210 : Product  Inputs=*/
  Divide_9a019 : Product  Inputs=*/
  Divide_afbf9 : Product  Inputs=*/
  MathFunc_cos_f109a : Trigonometry  Operator=cos
  MathFunc_sin_9f817 : Trigonometry
  Product_14786 : Product
  Product_14af6 : Product
  Product_1da26 : Product
  Product_34abd : Product
  Product_58aa4 : Product
  Product_8082a : Product
  Product_85ebc : Product
  Product_89931 : Product
  Product_af746 : Product
  Product_da8a8 : Product
  Product_ecfdc : Product
  Subtract_551ae : Sum  Inputs=+-
  Subtract_5e1fd : Sum  Inputs=+-
  Subtract_7015a : Sum  Inputs=+-
  Subtract_831c6 : Sum  Inputs=+-
  Subtract_8f742 : Sum  Inputs=+-
  Subtract_959a0 : Sum  Inputs=+-
  Subtract_f5459 : Sum  Inputs=+-
  Blockout_i_q_SG_D_1_7a201 : Outport
  wires:
  State_theta_SG_D_1_20748/1 -> MathFunc_cos_f109a/1
  State_psi_fd_SG_D_1_58d0e/1 -> Product_af746/1
  Constant_-1_a70be/1 -> Product_89931/1
  Constant_x_l_6df76/1 -> Product_89931/2
  Subtract_8f742/1 -> Product_af746/2
  Constant_x_l_111e7/1 -> Subtract_959a0/2
  Product_89931/1 -> Add_a0598/1
  Constant_x_qdd_0f738/1 -> Add_a0598/2
  Constant_x_qd_d5e1f/1 -> Subtract_5e1fd/1
  Constant_x_qdd_325a0/1 -> Divide_afbf9/2
  MathFunc_sin_9f817/1 -> Product_85ebc/2
  Constant_-1_41cb1/1 -> Product_14af6/1
  Constant_x_qdd_04085/1 -> Subtract_5e1fd/2
  Add_ee79c/1 -> Product_14786/2
  Product_8082a/1 -> Divide_9a019/1
  Constant_x_l_46464/1 -> Product_14af6/2
  Constant_-1_715c3/1 -> Product_da8a8/1
  Constant_x_l_3aa63/1 -> Product_da8a8/2
  State_psi_gq_SG_D_1_2717f/1 -> Product_8082a/1
  Add_a0598/1 -> Product_8082a/2
  Divide_58af2/1 -> Add_179e8/1
  Product_14af6/1 -> Add_2e471/1
  Divide_afbf9/1 -> Add_a475c/1
  Constant_x_qd_f127c/1 -> Add_2e471/2
  State_psi_kq_SG_D_1_bf4f0/1 -> Product_1da26/1
  Add_179e8/1 -> Subtract_7015a/1
  Subtract_5e1fd/1 -> Product_1da26/2
  Divide_9a019/1 -> Subtract_f5459/1
  Add_2e471/1 -> Divide_9a019/2
  Product_da8a8/1 -> Add_f0bd1/1
  Constant_x_qd_4819b/1 -> Add_f0bd1/2
  Constant_-1_3d43a/1 -> Product_ecfdc/1
  MathFunc_cos_f109a/1 -> Product_34abd/2
  Product_af746/1 -> Divide_663fd/1
  State_psi_1d_SG_D_1_d0628/1 -> Product_ecfdc/2
  Constant_x_l_cee03/1 -> Subtract_551ae/2
  Constant_x_dd_5089f/1 -> Subtract_831c6/1
  Divide_663fd/1 -> Subtract_7015a/2
  Constant_x_ddd_523dc/1 -> Subtract_831c6/2
  Product_34abd/1 -> Divide_86210/1
  Product_1da26/1 -> Divide_2e8ec/1
  Product_ecfdc/1 -> Product_58aa4/1
  Add_f0bd1/1 -> Divide_2e8ec/2
  Subtract_831c6/1 -> Product_58aa4/2
  State_psi_d_SG_D_1_d0c9d/1 -> Add_179e8/2
  Constant_x_dd_fe5f8/1 -> Subtract_959a0/1
  Constant_x_ddd_50ed9/1 -> Subtract_8f742/1
  Constant_x_l_81982/1 -> Subtract_8f742/2
  Divide_86210/1 -> Add_a475c/2
  Divide_2e8ec/1 -> Subtract_f5459/2
  State_theta_SG_D_1_baa8c/1 -> MathFunc_sin_9f817/1
  Product_58aa4/1 -> Divide_58af2/1
  Subtract_959a0/1 -> Divide_58af2/2
  Constant_x_dd_bd8fd/1 -> Subtract_551ae/1
  Subtract_f5459/1 -> Add_ee79c/1
  State_psi_q_SG_D_1_74a75/1 -> Add_ee79c/2
  Subtract_551ae/1 -> Divide_663fd/2
  Subtract_7015a/1 -> Product_34abd/1
  Constant_-1_8e5d6/1 -> Product_14786/1
  Product_14786/1 -> Product_85ebc/1
  Product_85ebc/1 -> Divide_afbf9/1
  Constant_x_ddd_2672a/1 -> Divide_86210/2
  Add_a475c/1 -> Blockout_i_q_SG_D_1_7a201/1

== system case4/SG_D_1/theta_SG_D_1_out_block ==
  note: theta_SG_D_1_out in case4
      | $\theta _{\mathrm{SG},D,1}$
      | Automatically generated on 2025-10-31 19:05:02 .
  State_theta_SG_D_1_0c8fe : Inport
  Blockout_theta_SG_D_1_out_ffb95 : Outport
  wires:
  State_theta_SG_D_1_0c8fe/1 -> Blockout_theta_SG_D_1_out_ffb95/1

== system case4/SG_D_1/w_SG_D_1_out_block ==
  note: w_SG_D_1_out in case4
      | $w_{\mathrm{SG},D,1}$
      | Automatically generated on 2025-10-31 19:05:02 .
  State_w_SG_D_1_a0747 : Inport
  Blockout_w_SG_D_1_out_8a23b : Outport
  wires:
  State_w_SG_D_1_a0747/1 -> Blockout_w_SG_D_1_out_8a23b/1
